simulink model "Transfert"  (Simulink 8.8)
settings: Solver=ode45  StartTime=0.0  StopTime=10.0  RelTol=1e-3  EnableMultiTasking=on
undefined symbols (not defined in the file or in its folder): Empattement, Voie
settings Model: SuppressorTable=22 serialization::archive 11 0 3 0 0 0 11 0  Creator=roland  LastModifiedBy=fnadi
settings OptimizationCC: ExpressionDepthLimit=2147483647  InitFltsAndDblsToZero=on
settings DebuggingCC: SolverPrmCheckMsg=warning  StrictBusMsg=Warning
settings HardwareCC: ProdHWDeviceType=Generic->Unspecified (assume 32-bit Generic)
settings GRTTargetCC: GeneratePreprocessorConditionals=Use local settings

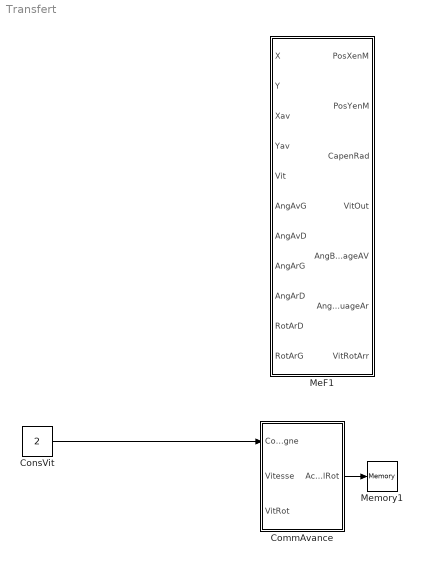
== system Transfert ==
  CommAvance : Subsystem
  ConsVit : Constant  Value=2
  MeF1 : Subsystem
  Memory1 : Memory  InheritSampleTime=on
  wires:
  CommAvance/1(AccelRot) -> Memory1/1
  ConsVit/1 -> CommAvance/1(Consigne)

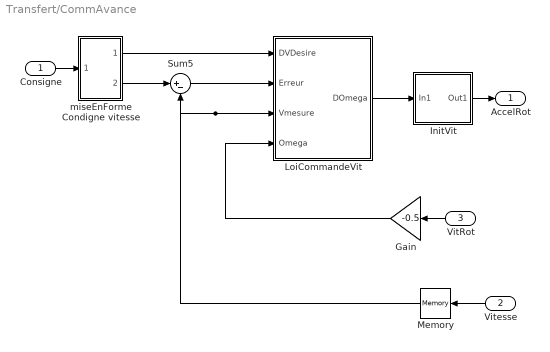
== system Transfert/CommAvance ==
  Consigne : Inport
  Vitesse : Inport  Port=2
  VitRot : Inport  Port=3
  Gain : Gain  Gain=-0.5  SaturateOnIntegerOverflow=on  OutDataTypeStr=Inherit: Same as input  ParamDataTypeStr=Inherit: Same as input
  InitVit : Subsystem
  LoiCommandeVit : Subsystem
  Memory : Memory  InheritSampleTime=on
  Sum5 : Sum  Inputs=|+-  SaturateOnIntegerOverflow=on
  miseEnForme Condigne vitesse : Subsystem
  AccelRot : Outport
  wires:
  LoiCommandeVit/1(DOmega) -> InitVit/1(In1)
  Sum5/1 -> LoiCommandeVit/2(Erreur)
  Gain/1 -> LoiCommandeVit/4(Omega)
  miseEnForme Condigne vitesse/2(Out2) -> Sum5/1
  miseEnForme Condigne vitesse/1(Out1) -> LoiCommandeVit/1(DVDesire)
  Memory/1 -> Sum5/2, LoiCommandeVit/3(Vmesure)
  Vitesse/1 -> Memory/1
  Consigne/1 -> miseEnForme Condigne vitesse/1(In1)
  InitVit/1(Out1) -> AccelRot/1
  VitRot/1 -> Gain/1

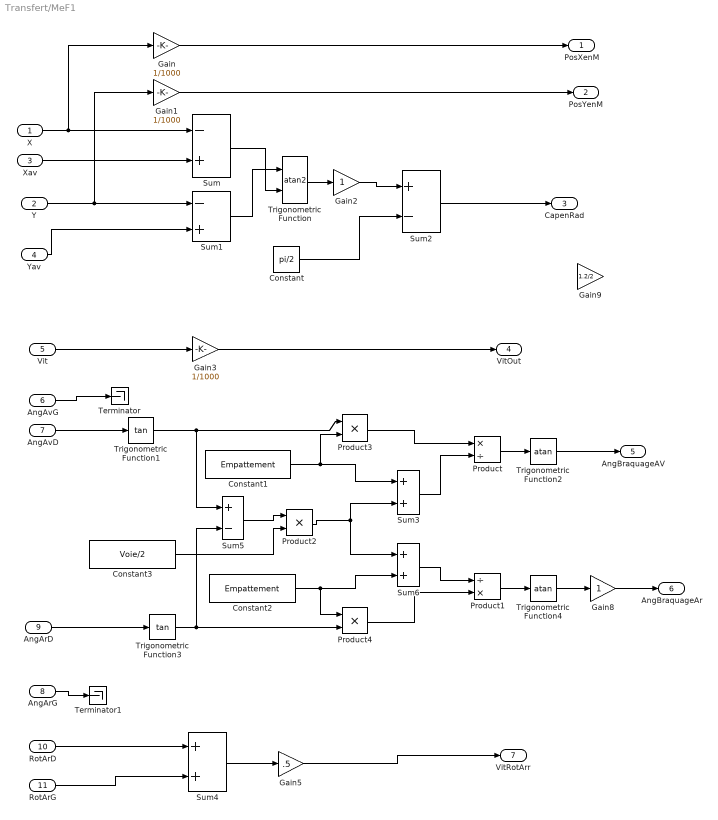
== system Transfert/MeF1 ==
  X : Inport
  Y : Inport  Port=2
  Xav : Inport  Port=3
  Yav : Inport  Port=4
  Vit : Inport  Port=5
  AngAvG : Inport  Port=6
  AngAvD : Inport  Port=7
  AngArG : Inport  Port=8
  AngArD : Inport  Port=9
  RotArD : Inport  Port=10
  RotArG : Inport  Port=11
  Constant : Constant  Value=pi/2
  Constant1 : Constant  Value=Empattement
  Constant2 : Constant  Value=Empattement
  Constant3 : Constant  Value=Voie/2
  Gain : Gain  Gain=1/1000
  Gain1 : Gain  Gain=1/1000
  Gain2 : Gain
  Gain3 : Gain  Gain=1/1000
  Gain5 : Gain  Gain=.5
  Gain8 : Gain
  Gain9 : Gain  Gain=1.2/2
  Product : Product  Inputs=*/  RndMeth=Zero
  Product1 : Product  Inputs=/*  RndMeth=Zero
  Product2 : Product  Inputs=**  RndMeth=Zero
  Product3 : Product  Inputs=**  RndMeth=Zero
  Product4 : Product  Inputs=**  RndMeth=Zero
  Sum : Sum  Inputs=-+
  Sum1 : Sum  Inputs=-+
  Sum2 : Sum  Inputs=+-
  Sum3 : Sum
  Sum4 : Sum
  Sum5 : Sum  Inputs=+-
  Sum6 : Sum
  Terminator : Terminator
  Terminator1 : Terminator
  Trigonometric Function : Trigonometry  Operator=atan2
  Trigonometric Function1 : Trigonometry  Operator=tan
  Trigonometric Function2 : Trigonometry  Operator=atan
  Trigonometric Function3 : Trigonometry  Operator=tan
  Trigonometric Function4 : Trigonometry  Operator=atan
  PosXenM : Outport
  PosYenM : Outport  Port=2
  CapenRad : Outport  Port=3
  VitOut : Outport  Port=4
  AngBraquageAV : Outport  Port=5
  AngBraquageAr : Outport  Port=6
  VitRotArr : Outport  Port=7
  wires:
  X/1 -> Sum/1, Gain/1
  Y/1 -> Sum1/1, Gain1/1
  Xav/1 -> Sum/2
  Trigonometric Function/1 -> Gain2/1
  Yav/1 -> Sum1/2
  Gain1/1 -> PosYenM/1
  Gain2/1 -> Sum2/1
  Constant/1 -> Sum2/2
  Sum2/1 -> CapenRad/1
  Vit/1 -> Gain3/1
  Gain3/1 -> VitOut/1
  AngAvD/1 -> Trigonometric Function1/1
  Sum4/1 -> Gain5/1
  RotArD/1 -> Sum4/1
  RotArG/1 -> Sum4/2
  Gain5/1 -> VitRotArr/1
  AngArD/1 -> Trigonometric Function3/1
  AngAvG/1 -> Terminator/1
  Trigonometric Function1/1 -> Sum5/1, Product3/1
  Sum3/1 -> Product/2
  Product3/1 -> Product/1
  Product/1 -> Trigonometric Function2/1
  Trigonometric Function2/1 -> AngBraquageAV/1
  AngArG/1 -> Terminator1/1
  Trigonometric Function3/1 -> Sum5/2, Product4/2
  Constant1/1 -> Sum3/1, Product3/2
  Sum5/1 -> Product2/1
  Product2/1 -> Sum3/2, Sum6/1
  Sum6/1 -> Product1/1
  Product4/1 -> Product1/2
  Constant2/1 -> Sum6/2, Product4/1
  Product1/1 -> Trigonometric Function4/1
  Trigonometric Function4/1 -> Gain8/1
  Gain8/1 -> AngBraquageAr/1
  Sum1/1 -> Trigonometric Function/1
  Sum/1 -> Trigonometric Function/2
  Gain/1 -> PosXenM/1
  Constant3/1 -> Product2/2

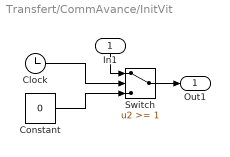
== system Transfert/CommAvance/InitVit ==
  In1 : Inport
  Clock : Clock
  Constant : Constant  Value=0
  Switch : Switch  Threshold=1  SaturateOnIntegerOverflow=on
  Out1 : Outport
  wires:
  Constant/1 -> Switch/3
  Clock/1 -> Switch/2
  In1/1 -> Switch/1
  Switch/1 -> Out1/1

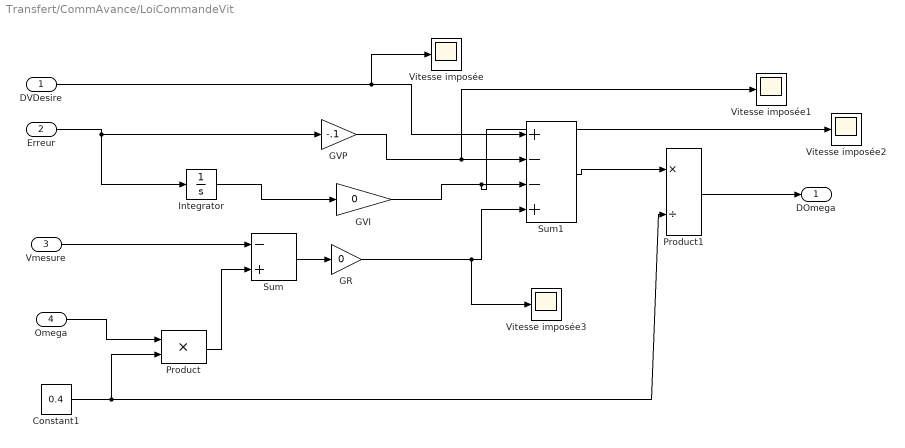
== system Transfert/CommAvance/LoiCommandeVit ==
  DVDesire : Inport
  Erreur : Inport  Port=2
  Vmesure : Inport  Port=3
  Omega : Inport  Port=4
  Constant1 : Constant  Value=0.4
  GR : Gain  Gain=0  SaturateOnIntegerOverflow=on  OutDataTypeStr=Inherit: Same as input  ParamDataTypeStr=Inherit: Same as input
  GVI : Gain  Gain=0  SaturateOnIntegerOverflow=on  OutDataTypeStr=Inherit: Same as input  ParamDataTypeStr=Inherit: Same as input
  GVP : Gain  Gain=-.1  SaturateOnIntegerOverflow=on  OutDataTypeStr=Inherit: Same as input  ParamDataTypeStr=Inherit: Same as input
  Integrator : Integrator
  Product : Product  SaturateOnIntegerOverflow=on  OutDataTypeStr=Inherit: Same as first input
  Product1 : Product  Inputs=*/  SaturateOnIntegerOverflow=on  OutDataTypeStr=Inherit: Same as first input
  Sum : Sum  Inputs=-+  SaturateOnIntegerOverflow=on
  Sum1 : Sum  Inputs=+--+  SaturateOnIntegerOverflow=on
  Vitesse imposée{,1..3} (4 alike) : Scope
  DOmega : Outport
  wires:
  GVI/1 -> Vitesse imposée2/1, Sum1/3
  GR/1 -> Sum1/4, Vitesse imposée3/1
  Product1/1 -> DOmega/1
  Sum1/1 -> Product1/1
  GVP/1 -> Vitesse imposée1/1, Sum1/2
  Erreur/1 -> GVP/1, Integrator/1
  DVDesire/1 -> Sum1/1, Vitesse imposée/1
  Sum/1 -> GR/1
  Vmesure/1 -> Sum/1
  Product/1 -> Sum/2
  Constant1/1 -> Product1/2, Product/2
  Omega/1 -> Product/1
  Integrator/1 -> GVI/1

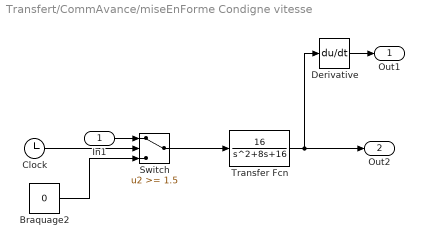
== system Transfert/CommAvance/miseEnForme Condigne vitesse ==
  In1 : Inport
  Braquage2 : Constant  Value=0
  Clock : Clock
  Derivative : Derivative
  Switch : Switch  Threshold=1.5
  Transfer Fcn : TransferFcn  Numerator=[16]  Denominator=[1 8 16]
  Out1 : Outport
  Out2 : Outport  Port=2
  wires:
  Transfer Fcn/1 -> Derivative/1, Out2/1
  Clock/1 -> Switch/2
  Braquage2/1 -> Switch/3
  Switch/1 -> Transfer Fcn/1
  Derivative/1 -> Out1/1
  In1/1 -> Switch/1
